simulink model "xEMU_SimulationModel3_rule1"  (R2017b)
settings: Solver=ode4  StartTime=0.0  StopTime=8192  FixedStep=0.01  RelTol=1e-3
undefined symbols (not defined in the file): a1, a2, a3, a4, ACO, BAT, Battery, DCT, DRT, EMS, ENV, Fahrzyklus_VS_modell, height_BAT, leistung, lib_bat, Maximum, Maximum_position, Num_cells, P_FC_max_long, P_FC_min_long, P_FC_step_max, Pbat_charge_max, Pbat_discharge_max, Pfc_max, Pfc_min, SOC_tar, time_peaks, TRM, velocity_peaks
libraries: simulink x5
(part 13 of 15)

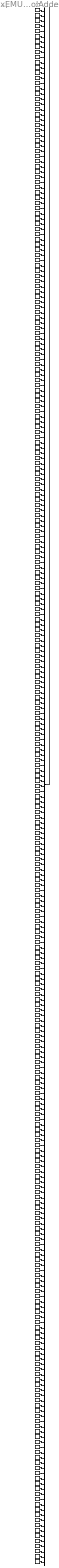
== system xEMU_SimulationModel3_rule1/Battery (BAT)_mittel/Subsystem1/Thermal/Coolings/CoolAdder ==
  P_cool : Inport
  Add_FV_{1..300} (300 alike) : Sum  Inputs=-
  Demux : Demux  Outputs=2
  Mux : Mux  Inputs=300
  P_FV : Outport
  wires:
  P_cool/1 -> Demux/1
  Mux/1 -> P_FV/1
  Add_FV_1/1 -> Mux/1
  Add_FV_2/1 -> Mux/2
  Add_FV_3/1 -> Mux/3
  Add_FV_4/1 -> Mux/4
  Add_FV_5/1 -> Mux/5
  Add_FV_6/1 -> Mux/6
  Add_FV_7/1 -> Mux/7
  Add_FV_8/1 -> Mux/8
  Add_FV_9/1 -> Mux/9
  Add_FV_10/1 -> Mux/10
  Add_FV_11/1 -> Mux/11
  Add_FV_12/1 -> Mux/12
  Add_FV_13/1 -> Mux/13
  Add_FV_14/1 -> Mux/14
  Add_FV_15/1 -> Mux/15
  Add_FV_16/1 -> Mux/16
  Add_FV_17/1 -> Mux/17
  Add_FV_18/1 -> Mux/18
  Add_FV_19/1 -> Mux/19
  Add_FV_20/1 -> Mux/20
  Add_FV_21/1 -> Mux/21
  Add_FV_22/1 -> Mux/22
  Add_FV_23/1 -> Mux/23
  Add_FV_24/1 -> Mux/24
  Add_FV_25/1 -> Mux/25
  Add_FV_26/1 -> Mux/26
  Add_FV_27/1 -> Mux/27
  Add_FV_28/1 -> Mux/28
  Add_FV_29/1 -> Mux/29
  Add_FV_30/1 -> Mux/30
  Add_FV_31/1 -> Mux/31
  Add_FV_32/1 -> Mux/32
  Add_FV_33/1 -> Mux/33
  Add_FV_34/1 -> Mux/34
  Add_FV_35/1 -> Mux/35
  Add_FV_36/1 -> Mux/36
  Add_FV_37/1 -> Mux/37
  Add_FV_38/1 -> Mux/38
  Add_FV_39/1 -> Mux/39
  Add_FV_40/1 -> Mux/40
  Add_FV_41/1 -> Mux/41
  Add_FV_42/1 -> Mux/42
  Add_FV_43/1 -> Mux/43
  Add_FV_44/1 -> Mux/44
  Add_FV_45/1 -> Mux/45
  Add_FV_46/1 -> Mux/46
  Add_FV_47/1 -> Mux/47
  Add_FV_48/1 -> Mux/48
  Add_FV_49/1 -> Mux/49
  Add_FV_50/1 -> Mux/50
  Add_FV_51/1 -> Mux/51
  Add_FV_52/1 -> Mux/52
  Add_FV_53/1 -> Mux/53
  Add_FV_54/1 -> Mux/54
  Add_FV_55/1 -> Mux/55
  Add_FV_56/1 -> Mux/56
  Add_FV_57/1 -> Mux/57
  Add_FV_58/1 -> Mux/58
  Add_FV_59/1 -> Mux/59
  Add_FV_60/1 -> Mux/60
  Add_FV_61/1 -> Mux/61
  Add_FV_62/1 -> Mux/62
  Add_FV_63/1 -> Mux/63
  Add_FV_64/1 -> Mux/64
  Add_FV_65/1 -> Mux/65
  Add_FV_66/1 -> Mux/66
  Add_FV_67/1 -> Mux/67
  Add_FV_68/1 -> Mux/68
  Add_FV_69/1 -> Mux/69
  Add_FV_70/1 -> Mux/70
  Add_FV_71/1 -> Mux/71
  Add_FV_72/1 -> Mux/72
  Add_FV_73/1 -> Mux/73
  Add_FV_74/1 -> Mux/74
  Add_FV_75/1 -> Mux/75
  Add_FV_76/1 -> Mux/76
  Add_FV_77/1 -> Mux/77
  Add_FV_78/1 -> Mux/78
  Add_FV_79/1 -> Mux/79
  Add_FV_80/1 -> Mux/80
  Add_FV_81/1 -> Mux/81
  Add_FV_82/1 -> Mux/82
  Add_FV_83/1 -> Mux/83
  Add_FV_84/1 -> Mux/84
  Add_FV_85/1 -> Mux/85
  Add_FV_86/1 -> Mux/86
  Add_FV_87/1 -> Mux/87
  Add_FV_88/1 -> Mux/88
  Add_FV_89/1 -> Mux/89
  Add_FV_90/1 -> Mux/90
  Add_FV_91/1 -> Mux/91
  Add_FV_92/1 -> Mux/92
  Add_FV_93/1 -> Mux/93
  Add_FV_94/1 -> Mux/94
  Add_FV_95/1 -> Mux/95
  Add_FV_96/1 -> Mux/96
  Add_FV_97/1 -> Mux/97
  Add_FV_98/1 -> Mux/98
  Add_FV_99/1 -> Mux/99
  Add_FV_100/1 -> Mux/100
  Add_FV_101/1 -> Mux/101
  Add_FV_102/1 -> Mux/102
  Add_FV_103/1 -> Mux/103
  Add_FV_104/1 -> Mux/104
  Add_FV_105/1 -> Mux/105
  Add_FV_106/1 -> Mux/106
  Add_FV_107/1 -> Mux/107
  Add_FV_108/1 -> Mux/108
  Add_FV_109/1 -> Mux/109
  Add_FV_110/1 -> Mux/110
  Add_FV_111/1 -> Mux/111
  Add_FV_112/1 -> Mux/112
  Add_FV_113/1 -> Mux/113
  Add_FV_114/1 -> Mux/114
  Add_FV_115/1 -> Mux/115
  Add_FV_116/1 -> Mux/116
  Add_FV_117/1 -> Mux/117
  Add_FV_118/1 -> Mux/118
  Add_FV_119/1 -> Mux/119
  Add_FV_120/1 -> Mux/120
  Add_FV_121/1 -> Mux/121
  Add_FV_122/1 -> Mux/122
  Add_FV_123/1 -> Mux/123
  Add_FV_124/1 -> Mux/124
  Add_FV_125/1 -> Mux/125
  Add_FV_126/1 -> Mux/126
  Add_FV_127/1 -> Mux/127
  Add_FV_128/1 -> Mux/128
  Add_FV_129/1 -> Mux/129
  Add_FV_130/1 -> Mux/130
  Add_FV_131/1 -> Mux/131
  Add_FV_132/1 -> Mux/132
  Add_FV_133/1 -> Mux/133
  Add_FV_134/1 -> Mux/134
  Add_FV_135/1 -> Mux/135
  Add_FV_136/1 -> Mux/136
  Add_FV_137/1 -> Mux/137
  Add_FV_138/1 -> Mux/138
  Add_FV_139/1 -> Mux/139
  Add_FV_140/1 -> Mux/140
  Add_FV_141/1 -> Mux/141
  Add_FV_142/1 -> Mux/142
  Add_FV_143/1 -> Mux/143
  Add_FV_144/1 -> Mux/144
  Add_FV_145/1 -> Mux/145
  Add_FV_146/1 -> Mux/146
  Add_FV_147/1 -> Mux/147
  Add_FV_148/1 -> Mux/148
  Add_FV_149/1 -> Mux/149
  Add_FV_150/1 -> Mux/150
  Add_FV_151/1 -> Mux/151
  Add_FV_152/1 -> Mux/152
  Add_FV_153/1 -> Mux/153
  Add_FV_154/1 -> Mux/154
  Add_FV_155/1 -> Mux/155
  Add_FV_156/1 -> Mux/156
  Add_FV_157/1 -> Mux/157
  Add_FV_158/1 -> Mux/158
  Add_FV_159/1 -> Mux/159
  Add_FV_160/1 -> Mux/160
  Add_FV_161/1 -> Mux/161
  Add_FV_162/1 -> Mux/162
  Add_FV_163/1 -> Mux/163
  Add_FV_164/1 -> Mux/164
  Add_FV_165/1 -> Mux/165
  Add_FV_166/1 -> Mux/166
  Add_FV_167/1 -> Mux/167
  Add_FV_168/1 -> Mux/168
  Add_FV_169/1 -> Mux/169
  Add_FV_170/1 -> Mux/170
  Add_FV_171/1 -> Mux/171
  Add_FV_172/1 -> Mux/172
  Add_FV_173/1 -> Mux/173
  Add_FV_174/1 -> Mux/174
  Add_FV_175/1 -> Mux/175
  Add_FV_176/1 -> Mux/176
  Add_FV_177/1 -> Mux/177
  Add_FV_178/1 -> Mux/178
  Add_FV_179/1 -> Mux/179
  Add_FV_180/1 -> Mux/180
  Add_FV_181/1 -> Mux/181
  Add_FV_182/1 -> Mux/182
  Add_FV_183/1 -> Mux/183
  Add_FV_184/1 -> Mux/184
  Add_FV_185/1 -> Mux/185
  Add_FV_186/1 -> Mux/186
  Add_FV_187/1 -> Mux/187
  Add_FV_188/1 -> Mux/188
  Add_FV_189/1 -> Mux/189
  Add_FV_190/1 -> Mux/190
  Add_FV_191/1 -> Mux/191
  Add_FV_192/1 -> Mux/192
  Add_FV_193/1 -> Mux/193
  Add_FV_194/1 -> Mux/194
  Add_FV_195/1 -> Mux/195
  Add_FV_196/1 -> Mux/196
  Add_FV_197/1 -> Mux/197
  Add_FV_198/1 -> Mux/198
  Add_FV_199/1 -> Mux/199
  Add_FV_200/1 -> Mux/200
  Add_FV_201/1 -> Mux/201
  Add_FV_202/1 -> Mux/202
  Add_FV_203/1 -> Mux/203
  Add_FV_204/1 -> Mux/204
  Add_FV_205/1 -> Mux/205
  Add_FV_206/1 -> Mux/206
  Add_FV_207/1 -> Mux/207
  Add_FV_208/1 -> Mux/208
  Add_FV_209/1 -> Mux/209
  Add_FV_210/1 -> Mux/210
  Add_FV_211/1 -> Mux/211
  Add_FV_212/1 -> Mux/212
  Add_FV_213/1 -> Mux/213
  Add_FV_214/1 -> Mux/214
  Add_FV_215/1 -> Mux/215
  Add_FV_216/1 -> Mux/216
  Add_FV_217/1 -> Mux/217
  Add_FV_218/1 -> Mux/218
  Add_FV_219/1 -> Mux/219
  Add_FV_220/1 -> Mux/220
  Add_FV_221/1 -> Mux/221
  Add_FV_222/1 -> Mux/222
  Add_FV_223/1 -> Mux/223
  Add_FV_224/1 -> Mux/224
  Add_FV_225/1 -> Mux/225
  Add_FV_226/1 -> Mux/226
  Add_FV_227/1 -> Mux/227
  Add_FV_228/1 -> Mux/228
  Add_FV_229/1 -> Mux/229
  Add_FV_230/1 -> Mux/230
  Add_FV_231/1 -> Mux/231
  Add_FV_232/1 -> Mux/232
  Add_FV_233/1 -> Mux/233
  Add_FV_234/1 -> Mux/234
  Add_FV_235/1 -> Mux/235
  Add_FV_236/1 -> Mux/236
  Add_FV_237/1 -> Mux/237
  Add_FV_238/1 -> Mux/238
  Add_FV_239/1 -> Mux/239
  Add_FV_240/1 -> Mux/240
  Add_FV_241/1 -> Mux/241
  Add_FV_242/1 -> Mux/242
  Add_FV_243/1 -> Mux/243
  Add_FV_244/1 -> Mux/244
  Add_FV_245/1 -> Mux/245
  Add_FV_246/1 -> Mux/246
  Add_FV_247/1 -> Mux/247
  Add_FV_248/1 -> Mux/248
  Add_FV_249/1 -> Mux/249
  Add_FV_250/1 -> Mux/250
  Add_FV_251/1 -> Mux/251
  Add_FV_252/1 -> Mux/252
  Add_FV_253/1 -> Mux/253
  Add_FV_254/1 -> Mux/254
  Add_FV_255/1 -> Mux/255
  Add_FV_256/1 -> Mux/256
  Add_FV_257/1 -> Mux/257
  Add_FV_258/1 -> Mux/258
  Add_FV_259/1 -> Mux/259
  Add_FV_260/1 -> Mux/260
  Add_FV_261/1 -> Mux/261
  Add_FV_262/1 -> Mux/262
  Add_FV_263/1 -> Mux/263
  Add_FV_264/1 -> Mux/264
  Add_FV_265/1 -> Mux/265
  Add_FV_266/1 -> Mux/266
  Add_FV_267/1 -> Mux/267
  Add_FV_268/1 -> Mux/268
  Add_FV_269/1 -> Mux/269
  Add_FV_270/1 -> Mux/270
  Add_FV_271/1 -> Mux/271
  Add_FV_272/1 -> Mux/272
  Add_FV_273/1 -> Mux/273
  Add_FV_274/1 -> Mux/274
  Add_FV_275/1 -> Mux/275
  Add_FV_276/1 -> Mux/276
  Add_FV_277/1 -> Mux/277
  Add_FV_278/1 -> Mux/278
  Add_FV_279/1 -> Mux/279
  Add_FV_280/1 -> Mux/280
  Add_FV_281/1 -> Mux/281
  Add_FV_282/1 -> Mux/282
  Add_FV_283/1 -> Mux/283
  Add_FV_284/1 -> Mux/284
  Add_FV_285/1 -> Mux/285
  Add_FV_286/1 -> Mux/286
  Add_FV_287/1 -> Mux/287
  Add_FV_288/1 -> Mux/288
  Add_FV_289/1 -> Mux/289
  Add_FV_290/1 -> Mux/290
  Add_FV_291/1 -> Mux/291
  Add_FV_292/1 -> Mux/292
  Add_FV_293/1 -> Mux/293
  Add_FV_294/1 -> Mux/294
  Add_FV_295/1 -> Mux/295
  Add_FV_296/1 -> Mux/296
  Add_FV_297/1 -> Mux/297
  Add_FV_298/1 -> Mux/298
  Add_FV_299/1 -> Mux/299
  Add_FV_300/1 -> Mux/300

== system xEMU_SimulationModel3_rule1/Battery (BAT)_mittel_02/Cell/ElectricalCircuit/SerialTwoPort_Elem1/Cellelement_Elem1 ==
  OhmicResistance_Elem4 : Subsystem
  ParallelRC_Elem1 : Subsystem
  ParallelRC_Elem2 : Subsystem
  ParallelRC_Elem3 : Subsystem
  SoC : Integrator  ExternalReset=rising  InitialCondition=SOC_tar*100  LimitOutput=on  UpperSaturationLimit=100  LowerSaturationLimit=0
  SoCFactor : Gain  Gain=0.0012077
  VoltageSource_Elem5 : Subsystem
  tag scope: SoC_CellElement1=global
  wires:
  [Reset] -> SoC/2
  SoC/1 -> OhmicResistance_Elem4/2(SoC), VoltageSource_Elem5/2(SoC), ParallelRC_Elem3/2(SoC), ParallelRC_Elem2/2(SoC), ParallelRC_Elem1/2(SoC), [SoC_CellElement1]
  [I_CellElement1] -> SoCFactor/1
  SoCFactor/1 -> SoC/1
  [T_CellElement1] -> OhmicResistance_Elem4/1(T), VoltageSource_Elem5/1(T), ParallelRC_Elem3/1(T), ParallelRC_Elem2/1(T), ParallelRC_Elem1/1(T)

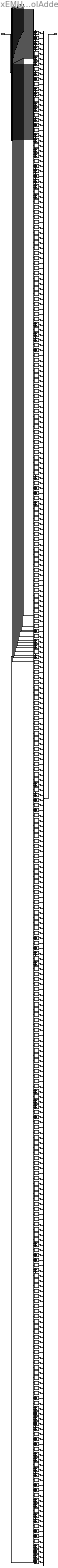
== system xEMU_SimulationModel3_rule1/Battery (BAT)_mittel_02/Cell/Thermal/Coolings/CoolAdder ==
  P_cool : Inport
  Add_FV_{1,3,28,30,271,273,298,300} (8 alike) : Sum  Inputs=+++
  Add_FV_{2,4,6..7,9..10,12..13,15..16,18..19,21..22,24..25,27,29,31,33,58,60..61,63,88,90..91,93,118,120..121,123,148,150..151,153,178,180..181,183,208,210..211,213,238,240..241,243,268,270,272,274,276..277,279..280,282..283,285..286,288..289,291..292,294..295,297,299} (68 alike) : Sum
  Add_FV_{5,8,11,14,17,20,23,26,32,34,36..37,39..40,42..43,45..46,48..49,51..52,54..55,57,59,62,64,66..67,69..70,72..73,75..76,78..79,81..82,84..85,87,89,92,94,96..97,99..100,102..103,105..106,108..109,111..112,114..115,117,119,122,124,126..127,129..130,132..133,135..136,138..139,141..142,144..145,147,149,152,154,156..157,159..160,162..163,165..166,168..169,171..172,174..175,177,179,182,184,186..187,189..190,192..193,195..196,198..199,201..202,204..205,207,209,212,214,216..217,219..220,222..223,225..226,228..229,231..232,234..235,237,239,242,244,246..247,249..250,252..253,255..256,258..259,261..262,264..265,267,269,275,278,281,284,287,290,293,296} (160 alike) : Sum  Inputs=+
  Add_FV_{35,38,41,44,47,50,53,56,65,68,71,74,77,80,83,86,95,98,101,104,107,110,113,116,125,128,131,134,137,140,143,146,155,158,161,164,167,170,173,176,185,188,191,194,197,200,203,206,215,218,221,224,227,230,233,236,245,248,251,254,257,260,263,266} (64 alike) : Sum  Inputs=-
  Demux : Demux  Outputs=320
  Mux : Mux  Inputs=300
  P_FV : Outport
  wires:
  P_cool/1 -> Demux/1
  Mux/1 -> P_FV/1
  Add_FV_1/1 -> Mux/1
  Add_FV_2/1 -> Mux/2
  Add_FV_3/1 -> Mux/3
  Add_FV_4/1 -> Mux/4
  Add_FV_5/1 -> Mux/5
  Add_FV_6/1 -> Mux/6
  Add_FV_7/1 -> Mux/7
  Add_FV_8/1 -> Mux/8
  Add_FV_9/1 -> Mux/9
  Add_FV_10/1 -> Mux/10
  Add_FV_11/1 -> Mux/11
  Add_FV_12/1 -> Mux/12
  Add_FV_13/1 -> Mux/13
  Add_FV_14/1 -> Mux/14
  Add_FV_15/1 -> Mux/15
  Add_FV_16/1 -> Mux/16
  Add_FV_17/1 -> Mux/17
  Add_FV_18/1 -> Mux/18
  Add_FV_19/1 -> Mux/19
  Add_FV_20/1 -> Mux/20
  Add_FV_21/1 -> Mux/21
  Add_FV_22/1 -> Mux/22
  Add_FV_23/1 -> Mux/23
  Add_FV_24/1 -> Mux/24
  Add_FV_25/1 -> Mux/25
  Add_FV_26/1 -> Mux/26
  Add_FV_27/1 -> Mux/27
  Add_FV_28/1 -> Mux/28
  Add_FV_29/1 -> Mux/29
  Add_FV_30/1 -> Mux/30
  Add_FV_31/1 -> Mux/31
  Add_FV_32/1 -> Mux/32
  Add_FV_33/1 -> Mux/33
  Add_FV_34/1 -> Mux/34
  Add_FV_35/1 -> Mux/35
  Add_FV_36/1 -> Mux/36
  Add_FV_37/1 -> Mux/37
  Add_FV_38/1 -> Mux/38
  Add_FV_39/1 -> Mux/39
  Add_FV_40/1 -> Mux/40
  Add_FV_41/1 -> Mux/41
  Add_FV_42/1 -> Mux/42
  Add_FV_43/1 -> Mux/43
  Add_FV_44/1 -> Mux/44
  Add_FV_45/1 -> Mux/45
  Add_FV_46/1 -> Mux/46
  Add_FV_47/1 -> Mux/47
  Add_FV_48/1 -> Mux/48
  Add_FV_49/1 -> Mux/49
  Add_FV_50/1 -> Mux/50
  Add_FV_51/1 -> Mux/51
  Add_FV_52/1 -> Mux/52
  Add_FV_53/1 -> Mux/53
  Add_FV_54/1 -> Mux/54
  Add_FV_55/1 -> Mux/55
  Add_FV_56/1 -> Mux/56
  Add_FV_57/1 -> Mux/57
  Add_FV_58/1 -> Mux/58
  Add_FV_59/1 -> Mux/59
  Add_FV_60/1 -> Mux/60
  Add_FV_61/1 -> Mux/61
  Add_FV_62/1 -> Mux/62
  Add_FV_63/1 -> Mux/63
  Add_FV_64/1 -> Mux/64
  Add_FV_65/1 -> Mux/65
  Add_FV_66/1 -> Mux/66
  Add_FV_67/1 -> Mux/67
  Add_FV_68/1 -> Mux/68
  Add_FV_69/1 -> Mux/69
  Add_FV_70/1 -> Mux/70
  Add_FV_71/1 -> Mux/71
  Add_FV_72/1 -> Mux/72
  Add_FV_73/1 -> Mux/73
  Add_FV_74/1 -> Mux/74
  Add_FV_75/1 -> Mux/75
  Add_FV_76/1 -> Mux/76
  Add_FV_77/1 -> Mux/77
  Add_FV_78/1 -> Mux/78
  Add_FV_79/1 -> Mux/79
  Add_FV_80/1 -> Mux/80
  Add_FV_81/1 -> Mux/81
  Add_FV_82/1 -> Mux/82
  Add_FV_83/1 -> Mux/83
  Add_FV_84/1 -> Mux/84
  Add_FV_85/1 -> Mux/85
  Add_FV_86/1 -> Mux/86
  Add_FV_87/1 -> Mux/87
  Add_FV_88/1 -> Mux/88
  Add_FV_89/1 -> Mux/89
  Add_FV_90/1 -> Mux/90
  Add_FV_91/1 -> Mux/91
  Add_FV_92/1 -> Mux/92
  Add_FV_93/1 -> Mux/93
  Add_FV_94/1 -> Mux/94
  Add_FV_95/1 -> Mux/95
  Add_FV_96/1 -> Mux/96
  Add_FV_97/1 -> Mux/97
  Add_FV_98/1 -> Mux/98
  Add_FV_99/1 -> Mux/99
  Add_FV_100/1 -> Mux/100
  Add_FV_101/1 -> Mux/101
  Add_FV_102/1 -> Mux/102
  Add_FV_103/1 -> Mux/103
  Add_FV_104/1 -> Mux/104
  Add_FV_105/1 -> Mux/105
  Add_FV_106/1 -> Mux/106
  Add_FV_107/1 -> Mux/107
  Add_FV_108/1 -> Mux/108
  Add_FV_109/1 -> Mux/109
  Add_FV_110/1 -> Mux/110
  Add_FV_111/1 -> Mux/111
  Add_FV_112/1 -> Mux/112
  Add_FV_113/1 -> Mux/113
  Add_FV_114/1 -> Mux/114
  Add_FV_115/1 -> Mux/115
  Add_FV_116/1 -> Mux/116
  Add_FV_117/1 -> Mux/117
  Add_FV_118/1 -> Mux/118
  Add_FV_119/1 -> Mux/119
  Add_FV_120/1 -> Mux/120
  Add_FV_121/1 -> Mux/121
  Add_FV_122/1 -> Mux/122
  Add_FV_123/1 -> Mux/123
  Add_FV_124/1 -> Mux/124
  Add_FV_125/1 -> Mux/125
  Add_FV_126/1 -> Mux/126
  Add_FV_127/1 -> Mux/127
  Add_FV_128/1 -> Mux/128
  Add_FV_129/1 -> Mux/129
  Add_FV_130/1 -> Mux/130
  Add_FV_131/1 -> Mux/131
  Add_FV_132/1 -> Mux/132
  Add_FV_133/1 -> Mux/133
  Add_FV_134/1 -> Mux/134
  Add_FV_135/1 -> Mux/135
  Add_FV_136/1 -> Mux/136
  Add_FV_137/1 -> Mux/137
  Add_FV_138/1 -> Mux/138
  Add_FV_139/1 -> Mux/139
  Add_FV_140/1 -> Mux/140
  Add_FV_141/1 -> Mux/141
  Add_FV_142/1 -> Mux/142
  Add_FV_143/1 -> Mux/143
  Add_FV_144/1 -> Mux/144
  Add_FV_145/1 -> Mux/145
  Add_FV_146/1 -> Mux/146
  Add_FV_147/1 -> Mux/147
  Add_FV_148/1 -> Mux/148
  Add_FV_149/1 -> Mux/149
  Add_FV_150/1 -> Mux/150
  Add_FV_151/1 -> Mux/151
  Add_FV_152/1 -> Mux/152
  Add_FV_153/1 -> Mux/153
  Add_FV_154/1 -> Mux/154
  Add_FV_155/1 -> Mux/155
  Add_FV_156/1 -> Mux/156
  Add_FV_157/1 -> Mux/157
  Add_FV_158/1 -> Mux/158
  Add_FV_159/1 -> Mux/159
  Add_FV_160/1 -> Mux/160
  Add_FV_161/1 -> Mux/161
  Add_FV_162/1 -> Mux/162
  Add_FV_163/1 -> Mux/163
  Add_FV_164/1 -> Mux/164
  Add_FV_165/1 -> Mux/165
  Add_FV_166/1 -> Mux/166
  Add_FV_167/1 -> Mux/167
  Add_FV_168/1 -> Mux/168
  Add_FV_169/1 -> Mux/169
  Add_FV_170/1 -> Mux/170
  Add_FV_171/1 -> Mux/171
  Add_FV_172/1 -> Mux/172
  Add_FV_173/1 -> Mux/173
  Add_FV_174/1 -> Mux/174
  Add_FV_175/1 -> Mux/175
  Add_FV_176/1 -> Mux/176
  Add_FV_177/1 -> Mux/177
  Add_FV_178/1 -> Mux/178
  Add_FV_179/1 -> Mux/179
  Add_FV_180/1 -> Mux/180
  Add_FV_181/1 -> Mux/181
  Add_FV_182/1 -> Mux/182
  Add_FV_183/1 -> Mux/183
  Add_FV_184/1 -> Mux/184
  Add_FV_185/1 -> Mux/185
  Add_FV_186/1 -> Mux/186
  Add_FV_187/1 -> Mux/187
  Add_FV_188/1 -> Mux/188
  Add_FV_189/1 -> Mux/189
  Add_FV_190/1 -> Mux/190
  Add_FV_191/1 -> Mux/191
  Add_FV_192/1 -> Mux/192
  Add_FV_193/1 -> Mux/193
  Add_FV_194/1 -> Mux/194
  Add_FV_195/1 -> Mux/195
  Add_FV_196/1 -> Mux/196
  Add_FV_197/1 -> Mux/197
  Add_FV_198/1 -> Mux/198
  Add_FV_199/1 -> Mux/199
  Add_FV_200/1 -> Mux/200
  Add_FV_201/1 -> Mux/201
  Add_FV_202/1 -> Mux/202
  Add_FV_203/1 -> Mux/203
  Add_FV_204/1 -> Mux/204
  Add_FV_205/1 -> Mux/205
  Add_FV_206/1 -> Mux/206
  Add_FV_207/1 -> Mux/207
  Add_FV_208/1 -> Mux/208
  Add_FV_209/1 -> Mux/209
  Add_FV_210/1 -> Mux/210
  Add_FV_211/1 -> Mux/211
  Add_FV_212/1 -> Mux/212
  Add_FV_213/1 -> Mux/213
  Add_FV_214/1 -> Mux/214
  Add_FV_215/1 -> Mux/215
  Add_FV_216/1 -> Mux/216
  Add_FV_217/1 -> Mux/217
  Add_FV_218/1 -> Mux/218
  Add_FV_219/1 -> Mux/219
  Add_FV_220/1 -> Mux/220
  Add_FV_221/1 -> Mux/221
  Add_FV_222/1 -> Mux/222
  Add_FV_223/1 -> Mux/223
  Add_FV_224/1 -> Mux/224
  Add_FV_225/1 -> Mux/225
  Add_FV_226/1 -> Mux/226
  Add_FV_227/1 -> Mux/227
  Add_FV_228/1 -> Mux/228
  Add_FV_229/1 -> Mux/229
  Add_FV_230/1 -> Mux/230
  Add_FV_231/1 -> Mux/231
  Add_FV_232/1 -> Mux/232
  Add_FV_233/1 -> Mux/233
  Add_FV_234/1 -> Mux/234
  Add_FV_235/1 -> Mux/235
  Add_FV_236/1 -> Mux/236
  Add_FV_237/1 -> Mux/237
  Add_FV_238/1 -> Mux/238
  Add_FV_239/1 -> Mux/239
  Add_FV_240/1 -> Mux/240
  Add_FV_241/1 -> Mux/241
  Add_FV_242/1 -> Mux/242
  Add_FV_243/1 -> Mux/243
  Add_FV_244/1 -> Mux/244
  Add_FV_245/1 -> Mux/245
  Add_FV_246/1 -> Mux/246
  Add_FV_247/1 -> Mux/247
  Add_FV_248/1 -> Mux/248
  Add_FV_249/1 -> Mux/249
  Add_FV_250/1 -> Mux/250
  Add_FV_251/1 -> Mux/251
  Add_FV_252/1 -> Mux/252
  Add_FV_253/1 -> Mux/253
  Add_FV_254/1 -> Mux/254
  Add_FV_255/1 -> Mux/255
  Add_FV_256/1 -> Mux/256
  Add_FV_257/1 -> Mux/257
  Add_FV_258/1 -> Mux/258
  Add_FV_259/1 -> Mux/259
  Add_FV_260/1 -> Mux/260
  Add_FV_261/1 -> Mux/261
  Add_FV_262/1 -> Mux/262
  Add_FV_263/1 -> Mux/263
  Add_FV_264/1 -> Mux/264
  Add_FV_265/1 -> Mux/265
  Add_FV_266/1 -> Mux/266
  Add_FV_267/1 -> Mux/267
  Add_FV_268/1 -> Mux/268
  Add_FV_269/1 -> Mux/269
  Add_FV_270/1 -> Mux/270
  Add_FV_271/1 -> Mux/271
  Add_FV_272/1 -> Mux/272
  Add_FV_273/1 -> Mux/273
  Add_FV_274/1 -> Mux/274
  Add_FV_275/1 -> Mux/275
  Add_FV_276/1 -> Mux/276
  Add_FV_277/1 -> Mux/277
  Add_FV_278/1 -> Mux/278
  Add_FV_279/1 -> Mux/279
  Add_FV_280/1 -> Mux/280
  Add_FV_281/1 -> Mux/281
  Add_FV_282/1 -> Mux/282
  Add_FV_283/1 -> Mux/283
  Add_FV_284/1 -> Mux/284
  Add_FV_285/1 -> Mux/285
  Add_FV_286/1 -> Mux/286
  Add_FV_287/1 -> Mux/287
  Add_FV_288/1 -> Mux/288
  Add_FV_289/1 -> Mux/289
  Add_FV_290/1 -> Mux/290
  Add_FV_291/1 -> Mux/291
  Add_FV_292/1 -> Mux/292
  Add_FV_293/1 -> Mux/293
  Add_FV_294/1 -> Mux/294
  Add_FV_295/1 -> Mux/295
  Add_FV_296/1 -> Mux/296
  Add_FV_297/1 -> Mux/297
  Add_FV_298/1 -> Mux/298
  Add_FV_299/1 -> Mux/299
  Add_FV_300/1 -> Mux/300
  Demux/1 -> Add_FV_1/1
  Demux/2 -> Add_FV_1/2
  Demux/3 -> Add_FV_1/3
  Demux/4 -> Add_FV_2/1
  Demux/5 -> Add_FV_2/2
  Demux/6 -> Add_FV_3/1
  Demux/7 -> Add_FV_3/2
  Demux/8 -> Add_FV_3/3
  Demux/9 -> Add_FV_4/1
  Demux/10 -> Add_FV_4/2
  Demux/11 -> Add_FV_5/1
  Demux/12 -> Add_FV_6/1
  Demux/13 -> Add_FV_6/2
  Demux/14 -> Add_FV_7/1
  Demux/15 -> Add_FV_7/2
  Demux/16 -> Add_FV_8/1
  Demux/17 -> Add_FV_9/1
  Demux/18 -> Add_FV_9/2
  Demux/19 -> Add_FV_10/1
  Demux/20 -> Add_FV_10/2
  Demux/21 -> Add_FV_11/1
  Demux/22 -> Add_FV_12/1
  Demux/23 -> Add_FV_12/2
  Demux/24 -> Add_FV_13/1
  Demux/25 -> Add_FV_13/2
  Demux/26 -> Add_FV_14/1
  Demux/27 -> Add_FV_15/1
  Demux/28 -> Add_FV_15/2
  Demux/29 -> Add_FV_16/1
  Demux/30 -> Add_FV_16/2
  Demux/31 -> Add_FV_17/1
  Demux/32 -> Add_FV_18/1
  Demux/33 -> Add_FV_18/2
  Demux/34 -> Add_FV_19/1
  Demux/35 -> Add_FV_19/2
  Demux/36 -> Add_FV_20/1
  Demux/37 -> Add_FV_21/1
  Demux/38 -> Add_FV_21/2
  Demux/39 -> Add_FV_22/1
  Demux/40 -> Add_FV_22/2
  Demux/41 -> Add_FV_23/1
  Demux/42 -> Add_FV_24/1
  Demux/43 -> Add_FV_24/2
  Demux/44 -> Add_FV_25/1
  Demux/45 -> Add_FV_25/2
  Demux/46 -> Add_FV_26/1
  Demux/47 -> Add_FV_27/1
  Demux/48 -> Add_FV_27/2
  Demux/49 -> Add_FV_28/1
  Demux/50 -> Add_FV_28/2
  Demux/51 -> Add_FV_28/3
  Demux/52 -> Add_FV_29/1
  Demux/53 -> Add_FV_29/2
  Demux/54 -> Add_FV_30/1
  Demux/55 -> Add_FV_30/2
  Demux/56 -> Add_FV_30/3
  Demux/57 -> Add_FV_31/1
  Demux/58 -> Add_FV_31/2
  Demux/59 -> Add_FV_32/1
  Demux/60 -> Add_FV_33/1
  Demux/61 -> Add_FV_33/2
  Demux/62 -> Add_FV_34/1
  Demux/63 -> Add_FV_36/1
  Demux/64 -> Add_FV_37/1
  Demux/65 -> Add_FV_39/1
  Demux/66 -> Add_FV_40/1
  Demux/67 -> Add_FV_42/1
  Demux/68 -> Add_FV_43/1
  Demux/69 -> Add_FV_45/1
  Demux/70 -> Add_FV_46/1
  Demux/71 -> Add_FV_48/1
  Demux/72 -> Add_FV_49/1
  Demux/73 -> Add_FV_51/1
  Demux/74 -> Add_FV_52/1
  Demux/75 -> Add_FV_54/1
  Demux/76 -> Add_FV_55/1
  Demux/77 -> Add_FV_57/1
  Demux/78 -> Add_FV_58/1
  Demux/79 -> Add_FV_58/2
  Demux/80 -> Add_FV_59/1
  Demux/81 -> Add_FV_60/1
  Demux/82 -> Add_FV_60/2
  Demux/83 -> Add_FV_61/1
  Demux/84 -> Add_FV_61/2
  Demux/85 -> Add_FV_62/1
  Demux/86 -> Add_FV_63/1
  Demux/87 -> Add_FV_63/2
  Demux/88 -> Add_FV_64/1
  Demux/89 -> Add_FV_66/1
  Demux/90 -> Add_FV_67/1
  Demux/91 -> Add_FV_69/1
  Demux/92 -> Add_FV_70/1
  Demux/93 -> Add_FV_72/1
  Demux/94 -> Add_FV_73/1
  Demux/95 -> Add_FV_75/1
  Demux/96 -> Add_FV_76/1
  Demux/97 -> Add_FV_78/1
  Demux/98 -> Add_FV_79/1
  Demux/99 -> Add_FV_81/1
  Demux/100 -> Add_FV_82/1
  Demux/101 -> Add_FV_84/1
  Demux/102 -> Add_FV_85/1
  Demux/103 -> Add_FV_87/1
  Demux/104 -> Add_FV_88/1
  Demux/105 -> Add_FV_88/2
  Demux/106 -> Add_FV_89/1
  Demux/107 -> Add_FV_90/1
  Demux/108 -> Add_FV_90/2
  Demux/109 -> Add_FV_91/1
  Demux/110 -> Add_FV_91/2
  Demux/111 -> Add_FV_92/1
  Demux/112 -> Add_FV_93/1
  Demux/113 -> Add_FV_93/2
  Demux/114 -> Add_FV_94/1
  Demux/115 -> Add_FV_96/1
  Demux/116 -> Add_FV_97/1
  Demux/117 -> Add_FV_99/1
  Demux/118 -> Add_FV_100/1
  Demux/119 -> Add_FV_102/1
  Demux/120 -> Add_FV_103/1
  Demux/121 -> Add_FV_105/1
  Demux/122 -> Add_FV_106/1
  Demux/123 -> Add_FV_108/1
  Demux/124 -> Add_FV_109/1
  Demux/125 -> Add_FV_111/1
  Demux/126 -> Add_FV_112/1
  Demux/127 -> Add_FV_114/1
  Demux/128 -> Add_FV_115/1
  Demux/129 -> Add_FV_117/1
  Demux/130 -> Add_FV_118/1
  Demux/131 -> Add_FV_118/2
  Demux/132 -> Add_FV_119/1
  Demux/133 -> Add_FV_120/1
  Demux/134 -> Add_FV_120/2
  Demux/135 -> Add_FV_121/1
  Demux/136 -> Add_FV_121/2
  Demux/137 -> Add_FV_122/1
  Demux/138 -> Add_FV_123/1
  Demux/139 -> Add_FV_123/2
  Demux/140 -> Add_FV_124/1
  Demux/141 -> Add_FV_126/1
  Demux/142 -> Add_FV_127/1
  Demux/143 -> Add_FV_129/1
  Demux/144 -> Add_FV_130/1
  Demux/145 -> Add_FV_132/1
  Demux/146 -> Add_FV_133/1
  Demux/147 -> Add_FV_135/1
  Demux/148 -> Add_FV_136/1
  Demux/149 -> Add_FV_138/1
  Demux/150 -> Add_FV_139/1
  Demux/151 -> Add_FV_141/1
  Demux/152 -> Add_FV_142/1
  Demux/153 -> Add_FV_144/1
  Demux/154 -> Add_FV_145/1
  Demux/155 -> Add_FV_147/1
  Demux/156 -> Add_FV_148/1
  Demux/157 -> Add_FV_148/2
  Demux/158 -> Add_FV_149/1
  Demux/159 -> Add_FV_150/1
  Demux/160 -> Add_FV_150/2
  Demux/161 -> Add_FV_151/1
  Demux/162 -> Add_FV_151/2
  Demux/163 -> Add_FV_152/1
  Demux/164 -> Add_FV_153/1
  Demux/165 -> Add_FV_153/2
  Demux/166 -> Add_FV_154/1
  Demux/167 -> Add_FV_156/1
  Demux/168 -> Add_FV_157/1
  Demux/169 -> Add_FV_159/1
  Demux/170 -> Add_FV_160/1
  Demux/171 -> Add_FV_162/1
  Demux/172 -> Add_FV_163/1
  Demux/173 -> Add_FV_165/1
  Demux/174 -> Add_FV_166/1
  Demux/175 -> Add_FV_168/1
  Demux/176 -> Add_FV_169/1
  Demux/177 -> Add_FV_171/1
  Demux/178 -> Add_FV_172/1
  Demux/179 -> Add_FV_174/1
  Demux/180 -> Add_FV_175/1
  Demux/181 -> Add_FV_177/1
  Demux/182 -> Add_FV_178/1
  Demux/183 -> Add_FV_178/2
  Demux/184 -> Add_FV_179/1
  Demux/185 -> Add_FV_180/1
  Demux/186 -> Add_FV_180/2
  Demux/187 -> Add_FV_181/1
  Demux/188 -> Add_FV_181/2
  Demux/189 -> Add_FV_182/1
  Demux/190 -> Add_FV_183/1
  Demux/191 -> Add_FV_183/2
  Demux/192 -> Add_FV_184/1
  Demux/193 -> Add_FV_186/1
  Demux/194 -> Add_FV_187/1
  Demux/195 -> Add_FV_189/1
  Demux/196 -> Add_FV_190/1
  Demux/197 -> Add_FV_192/1
  Demux/198 -> Add_FV_193/1
  Demux/199 -> Add_FV_195/1
  Demux/200 -> Add_FV_196/1
  Demux/201 -> Add_FV_198/1
  Demux/202 -> Add_FV_199/1
  Demux/203 -> Add_FV_201/1
  Demux/204 -> Add_FV_202/1
  Demux/205 -> Add_FV_204/1
  Demux/206 -> Add_FV_205/1
  Demux/207 -> Add_FV_207/1
  Demux/208 -> Add_FV_208/1
  Demux/209 -> Add_FV_208/2
  Demux/210 -> Add_FV_209/1
  Demux/211 -> Add_FV_210/1
  Demux/212 -> Add_FV_210/2
  Demux/213 -> Add_FV_211/1
  Demux/214 -> Add_FV_211/2
  Demux/215 -> Add_FV_212/1
  Demux/216 -> Add_FV_213/1
  Demux/217 -> Add_FV_213/2
  Demux/218 -> Add_FV_214/1
  Demux/219 -> Add_FV_216/1
  Demux/220 -> Add_FV_217/1
  Demux/221 -> Add_FV_219/1
  Demux/222 -> Add_FV_220/1
  Demux/223 -> Add_FV_222/1
  Demux/224 -> Add_FV_223/1
  Demux/225 -> Add_FV_225/1
  Demux/226 -> Add_FV_226/1
  Demux/227 -> Add_FV_228/1
  Demux/228 -> Add_FV_229/1
  Demux/229 -> Add_FV_231/1
  Demux/230 -> Add_FV_232/1
  Demux/231 -> Add_FV_234/1
  Demux/232 -> Add_FV_235/1
  Demux/233 -> Add_FV_237/1
  Demux/234 -> Add_FV_238/1
  Demux/235 -> Add_FV_238/2
  Demux/236 -> Add_FV_239/1
  Demux/237 -> Add_FV_240/1
  Demux/238 -> Add_FV_240/2
  Demux/239 -> Add_FV_241/1
  Demux/240 -> Add_FV_241/2
  Demux/241 -> Add_FV_242/1
  Demux/242 -> Add_FV_243/1
  Demux/243 -> Add_FV_243/2
  Demux/244 -> Add_FV_244/1
  Demux/245 -> Add_FV_246/1
  Demux/246 -> Add_FV_247/1
  Demux/247 -> Add_FV_249/1
  Demux/248 -> Add_FV_250/1
  Demux/249 -> Add_FV_252/1
  Demux/250 -> Add_FV_253/1
  Demux/251 -> Add_FV_255/1
  Demux/252 -> Add_FV_256/1
  Demux/253 -> Add_FV_258/1
  Demux/254 -> Add_FV_259/1
  Demux/255 -> Add_FV_261/1
  Demux/256 -> Add_FV_262/1
  Demux/257 -> Add_FV_264/1
  Demux/258 -> Add_FV_265/1
  Demux/259 -> Add_FV_267/1
  Demux/260 -> Add_FV_268/1
  Demux/261 -> Add_FV_268/2
  Demux/262 -> Add_FV_269/1
  Demux/263 -> Add_FV_270/1
  Demux/264 -> Add_FV_270/2
  Demux/265 -> Add_FV_271/1
  Demux/266 -> Add_FV_271/2
  Demux/267 -> Add_FV_271/3
  Demux/268 -> Add_FV_272/1
  Demux/269 -> Add_FV_272/2
  Demux/270 -> Add_FV_273/1
  Demux/271 -> Add_FV_273/2
  Demux/272 -> Add_FV_273/3
  Demux/273 -> Add_FV_274/1
  Demux/274 -> Add_FV_274/2
  Demux/275 -> Add_FV_275/1
  Demux/276 -> Add_FV_276/1
  Demux/277 -> Add_FV_276/2
  Demux/278 -> Add_FV_277/1
  Demux/279 -> Add_FV_277/2
  Demux/280 -> Add_FV_278/1
  Demux/281 -> Add_FV_279/1
  Demux/282 -> Add_FV_279/2
  Demux/283 -> Add_FV_280/1
  Demux/284 -> Add_FV_280/2
  Demux/285 -> Add_FV_281/1
  Demux/286 -> Add_FV_282/1
  Demux/287 -> Add_FV_282/2
  Demux/288 -> Add_FV_283/1
  Demux/289 -> Add_FV_283/2
  Demux/290 -> Add_FV_284/1
  Demux/291 -> Add_FV_285/1
  Demux/292 -> Add_FV_285/2
  Demux/293 -> Add_FV_286/1
  Demux/294 -> Add_FV_286/2
  Demux/295 -> Add_FV_287/1
  Demux/296 -> Add_FV_288/1
  Demux/297 -> Add_FV_288/2
  Demux/298 -> Add_FV_289/1
  Demux/299 -> Add_FV_289/2
  Demux/300 -> Add_FV_290/1
  Demux/301 -> Add_FV_291/1
  Demux/302 -> Add_FV_291/2
  Demux/303 -> Add_FV_292/1
  Demux/304 -> Add_FV_292/2
  Demux/305 -> Add_FV_293/1
  Demux/306 -> Add_FV_294/1
  Demux/307 -> Add_FV_294/2
  Demux/308 -> Add_FV_295/1
  Demux/309 -> Add_FV_295/2
  Demux/310 -> Add_FV_296/1
  Demux/311 -> Add_FV_297/1
  Demux/312 -> Add_FV_297/2
  Demux/313 -> Add_FV_298/1
  Demux/314 -> Add_FV_298/2
  Demux/315 -> Add_FV_298/3
  Demux/316 -> Add_FV_299/1
  Demux/317 -> Add_FV_299/2
  Demux/318 -> Add_FV_300/1
  Demux/319 -> Add_FV_300/2
  Demux/320 -> Add_FV_300/3

== system xEMU_SimulationModel3_rule1/Battery (BAT)_mittel_02/Cell/Thermal/Coolings/DefaultCooling_Elem1 ==
  T_FV : Inport
  Add : Sum
  Add1 : Sum
  Areas : Gain  Gain=[8.50666666666667e-05;7.77333333333333e-05;0.00012296;8.50666666666667e-05;7.77333333333333e-05;8.50666666666667e-05;7.77333333333333e-05;0.00012296;8.50666666666667e-05;0.00012296;8.50666666666667e-05;8.50666666666667e-05;0.00012296;8.50666666666667e-05;0.00012296;8.50666666666667e-05;8.50666666666667e-05;0.00012296;8.50666666666667e-05;0.00012296;8.50666666666667e-05;8.50666666666667e-05;0.00012296;8.50666666666667e-05;0.00012296;8.50666666666667e-05;8.50666666666667e-05;0.00012296;8.50666666666667e-05;0.00012296;8.50666666666667e-05;8.50666666666667e-05;0.00012296;8.50666666666667e-05;0.00012296;8.50666666666667e-05;8.50666666666667e-05;0.00012296;8.50666666666667e-05;0.00012296;8.50666666666667e-05;8.50666666666667e-05;0.00012296;8.50666666666667e-05;0.00012296;8.50666666666667e-05;8.50666666666667e-05;0.00012296;8.50666666666667e-05;7.77333333333333e-05;0.00012296;8.50666666666667e-05;7.77333333333333e-05;8.50666666666667e-05;7.77333333333333e-05;0.00012296;7.77333333333333e-05;0.00012296;7.77333333333333e-05;7.77333333333333e-05;0.00012296;0.00012296;0.00012296;0.00012296;0.00012296;0.00012296;0.00012296;0.00012296;0.00012296;0.00012296;0.00012296;0.00012296;0.00012296;0.00012296;0.00012296;0.00012296;0.00012296;7.77333333333333e-05;0.00012296;7.77333333333333e-05;7.77333333333333e-05;0.00012296;7.77333333333333e-05;0.00012296;7.77333333333333e-05;7.77333333333333e-05;0.00012296;0.00012296;0.00012296;0.00012296;0.00012296;0.00012296;0.00012296;0.00012296;0.00012296;0.00012296;0.00012296;0.00012296;0.00012296;0.00012296;0.00012296;0.00012296;0.00012296;7.77333333333333e-05;0.00012296;7.77333333333333e-05;7.77333333333333e-05;0.00012296;7.77333333333333e-05;0.00012296;7.77333333333333e-05;7.77333333333333e-05;0.00012296;0.00012296;0.00012296;0.00012296;0.00012296;0.00012296;0.00012296;0.00012296;0.00012296;0.00012296;0.00012296;0.00012296;0.00012296;0.00012296;0.00012296;0.00012296;0.00012296;7.77333333333333e-05;0.00012296;7.77333333333333e-05;7.77333333333333e-05;0.00012296;7.77333333333333e-05;0.00012296;7.77333333333333e-05;7.77333333333333e-05;0.00012296;0.00012296;0.00012296;0.00012296;0.00012296;0.00012296;0.00012296;0.00012296;0.00012296;0.00012296;0.00012296;0.00012296;0.00012296;0.00012296;0.00012296;0.00012296;0.00012296;7.77333333333333e-05;0.00012296;7.77333333333333e-05;7.77333333333333e-05;0.00012296;7.77333333333333e-05;0.00012296;7.77333333333333e-05;7.77333333333333e-05;0.00012296;0.00012296;0.00012296;0.00012296;0.00012296;0.00012296;0.00012296;0.00012296;0.00012296;0.00012296;0.00012296;0.00012296;0.00012296;0.00012296;0.00012296;0.00012296;0.00012296;7.77333333333333e-05;0.00012296;7.77333333333333e-05;7.77333333333333e-05;0.00012296;7.77333333333333e-05;0.00012296;7.77333333333333e-05;7.77333333333333e-05;0.00012296;0.00012296;0.00012296;0.00012296;0.00012296;0.00012296;0.00012296;0.00012296;0.00012296;0.00012296;0.00012296;0.00012296;0.00012296;0.00012296;0.00012296;0.00012296;0.00012296;7.77333333333333e-05;0.00012296;7.77333333333333e-05;7.77333333333333e-05;0.00012296;7.77333333333333e-05;0.00012296;7.77333333333333e-05;7.77333333333333e-05;0.00012296;0.00012296;0.00012296;0.00012296;0.00012296;0.00012296;0.00012296;0.00012296;0.00012296;0.00012296;0.00012296;0.00012296;0.00012296;0.00012296;0.00012296;0.00012296;0.00012296;7.77333333333333e-05;0.00012296;7.77333333333333e-05;7.77333333333333e-05;0.00012296;7.77333333333333e-05;0.00012296;7.77333333333333e-05;7.77333333333333e-05;0.00012296;0.00012296;0.00012296;0.00012296;0.00012296;0.00012296;0.00012296;0.00012296;0.00012296;0.00012296;0.00012296;0.00012296;0.00012296;0.00012296;0.00012296;0.00012296;0.00012296;7.77333333333333e-05;0.00012296;7.77333333333333e-05;7.77333333333333e-05;0.00012296;8.50666666666667e-05;7.77333333333333e-05;0.00012296;8.50666666666667e-05;7.77333333333333e-05;8.50666666666667e-05;7.77333333333333e-05;0.00012296;8.50666666666667e-05;0.00012296;8.50666666666667e-05;8.50666666666667e-05;0.00012296;8.50666666666667e-05 ...(+722 chars)]
  CelsiusToKelvin : Constant  Value=273.15
  DefaultCooling : MATLAB Function  TreatAsAtomicUnit=on
  Selector : Selector  InputPortWidth=300  IndexOptions=Index vector (dialog)  Indices=[1 1 1 2 2 3 3 3 4 4 5 6 6 7 7 8 9 9 10 10 11 12 12 13 13 14 15 15 16 16 17 18 18 19 19 20 21 21 22 22 23 24 24 25 25 26 27 27 28 28 28 29 29 30 30 30 31 31 32 33 33 34 36 37 39 40 42 43 45 46 48 49 51 52 54 55 57 58 58 59 60 60 61 61 62 63 63 64 66 67 69 70 72 73 75 76 78 79 81 82 84 85 87 88 88 89 90 90 91 91 92 93 93 94 96 97 99 100 102 103 105 106 108 109 111 112 114 115 117 118 118 119 120 120 121 121 122 123 123 124 126 127 129 130 132 133 135 136 138 139 141 142 144 145 147 148 148 149 150 150 151 151 152 153 153 154 156 157 159 160 162 163 165 166 168 169 171 172 174 175 177 178 178 179 180 180 181 181 182 183 183 184 186 187 189 190 192 193 195 196 198 199 201 202 204 205 207 208 208 209 210 210 211 211 212 213 213 214 216 217 219 220 222 223 225 226 228 229 231 232 234 235 237 238 238 239 240 240 241 241 242 243 243 244 246 247 249 250 252 253 255 256 258 259 261 262 264 265 267 268 268 269 270 270 271 271 271 272 272 273 273 273 274 274 275 276 276 277 277 278 279 279 280 280 281 282 282 283 283 284 285 285 286 286 287 288 288 289 289 290 291 291 292 292 293 294 294 295 295 296 297 297 298 298 298 299 299 300 300 300]  OutputSizes=1
  P_cool : Outport
  wires:
  [AirTemperature] -> Add1/2
  Add1/1 -> DefaultCooling/2(airTemperature)
  CelsiusToKelvin/1 -> Add/2, Add1/1
  Areas/1 -> P_cool/1
  DefaultCooling/1(y) -> Areas/1
  Add/1 -> DefaultCooling/1(u)
  Selector/1 -> Add/1
  T_FV/1 -> Selector/1

== system xEMU_SimulationModel3_rule1/Drive Train (DRT)/Slipmodel and Traction /Variant Subsystem1/Mit_Schlupf_nach_Kalker/Slip Model ==
  note: gradient of tangential stress
  note: Tangential Force Fx=2*Fz*u/pi*(E/(1+E^2)+atan(E))
      |
      | gradient of tangential stress E=G*pi*a*b*C11*S/Fz/u/4
  Fz_tire : Inport
  slip : Inport  Port=2
  adhesion : Inport  Port=3
  " " : Fcn  Expr=u/(1+u^2)+atan(u)
  Divide : Product  Inputs=/*/
  Gain : Gain  Gain=Schub_drt*pi*a_drt*b_drt*C11_drt/4
  Gain1 : Gain  Gain=2/pi
  Product : Product  Inputs=3
  f_traction_tire : Outport
  wires:
  " "/1 -> Gain1/1
  Divide/1 -> " "/1
  Product/1 -> f_traction_tire/1
  Gain1/1 -> Product/2
  adhesion/1 -> Divide/3, Product/3
  Fz_tire/1 -> Divide/1, Product/1
  Gain/1 -> Divide/2
  slip/1 -> Gain/1

== system xEMU_SimulationModel3_rule1/Drive Train (DRT)/Slipmodel and Traction /Variant Subsystem1/Mit_Schlupf_nach_Kalker/Tire Dynamics ==
  Resistance of tire : Inport
  T_EMAdemandper_axis_Nm : Inport  Port=2
  v_train_m/s : Inport  Port=3
  Abs1 : Abs
  Abs2 : Abs
  Constant : Constant  Value=eps
  Gain : Gain  Gain=1/2
  Gain1 : Gain  Gain=1/J_drt
  Gain2 : Gain  Gain=R_wheel_drt_m
  Gain3 : Gain  Gain=1/50
  Integrator : Integrator  LowerSaturationLimit=0
  Integrator1 : Integrator
  MATLAB Function : MATLAB Function  TreatAsAtomicUnit=on
  MATLAB Function1 : MATLAB Function  TreatAsAtomicUnit=on
  Max : MinMax  Function=max  Inputs=3
  Product : Product
  Relay : Relay  OnSwitchValue=0.3  OffSwitchValue=0.01
  Relay1 : Relay  OnSwitchValue=0.2  OffSwitchValue=0.01
  Saturation : Saturate  UpperLimit=1  LowerLimit=-1
  Saturation2 : Saturate  UpperLimit=inf  LowerLimit=0
  Scope9 : Scope
  Subtract : Sum  Inputs=+-
  Subtract1 : Sum  Inputs=+-
  Sum : Sum  Inputs=-+|
  Switch : Switch  Criteria=u2 > Threshold
  slip : Outport
  WheelSpeed_rad/s : Outport  Port=2
  wires:
  MATLAB Function/1(s) -> Saturation/1
  Integrator/1 -> Saturation2/1  "ohneFilter"
  Constant/1 -> Max/3
  Abs2/1 -> Product/1, Max/2
  Abs1/1 -> Max/1
  Saturation/1 -> Switch/1  "Kalker"
  Sum/1 -> Gain1/1
  Max/1 -> MATLAB Function/2(v)
  Subtract/1 -> Subtract1/1, MATLAB Function/1(dv)
  Gain1/1 -> Integrator/1
  Gain2/1 -> Subtract/1, Abs1/1
  T_EMAdemandper_axis_Nm/1 -> Gain/1
  Gain/1 -> Sum/2
  Resistance of tire/1 -> Sum/1
  Product/1 -> Subtract1/2
  Subtract1/1 -> Gain3/1
  Gain3/1 -> Integrator1/1
  Integrator1/1 -> Switch/3, Product/2  "Dampf"
  Switch/1 -> slip/1
  v_train_m/s/1 -> Scope9/1, Relay1/1, Subtract/2, Abs2/1
  Saturation2/1 -> Gain2/1, Relay/1, WheelSpeed_rad/s/1
  Relay/1 -> Switch/2

== system xEMU_SimulationModel3_rule1/Drive Train (DRT)/Slipmodel and Traction /Variant Subsystem1/Mit_Schlupf_nach_Yoshiki/Slip Model ==
  note: Tangential Force Fx=Fz*u
      |
      | friction coefficient u=c*exp(-a*s)-d*exp(-b*s)
  Fz_tire : Inport
  slip_speed : Inport  Port=2
  adhesionCoefficient_abs : Inport  Port=3
  wheelspeed : Inport  Port=4
  " " : Fcn  Expr=1*exp(-0.54*u(1))-1*exp(-1.2*u(1))
  MATLAB Function1 : MATLAB Function  TreatAsAtomicUnit=on
  Product : Product
  Scope : Scope
  f_traction_tire : Outport
  wires:
  " "/1 -> MATLAB Function1/1(ad_factor)
  Fz_tire/1 -> Product/1
  slip_speed/1 -> " "/1
  [v_ist] -> MATLAB Function1/4(v_ist)
  [v_soll] -> MATLAB Function1/5(v_soll)
  Product/1 -> f_traction_tire/1
  adhesionCoefficient_abs/1 -> MATLAB Function1/2(ad_rail)
  MATLAB Function1/1(ad_factor_final) -> Product/2
  wheelspeed/1 -> Scope/1, MATLAB Function1/3(w)

== system xEMU_SimulationModel3_rule1/Drive Train (DRT)/Slipmodel and Traction /Variant Subsystem1/Mit_Schlupf_nach_Yoshiki/Tire Dynamics ==
  note: w
  Resistance of tire : Inport
  T_EMAdemandper_axis_Nm : Inport  Port=2
  v_train_m/s : Inport  Port=3
  Abs1 : Abs
  Abs2 : Abs
  Constant : Constant  Value=eps
  Gain : Gain  Gain=1/2
  Gain1 : Gain  Gain=1/J_drt
  Gain2 : Gain  Gain=R_wheel_drt_m
  Integrator : Integrator  LimitOutput=on  LowerSaturationLimit=0
  MATLAB Function : MATLAB Function  TreatAsAtomicUnit=on
  MATLAB Function1 : MATLAB Function  TreatAsAtomicUnit=on
  Max : MinMax  Function=max  Inputs=3
  Saturation : Saturate  UpperLimit=1  LowerLimit=-1
  Subtract : Sum  Inputs=+-
  Sum : Sum  Inputs=-+|
  slip : Scope
  slip_speed : Outport
  WheelSpeed_rad/s : Outport  Port=2
  wires:
  MATLAB Function/1(s) -> Saturation/1
  Constant/1 -> Max/3
  Abs2/1 -> Max/2
  Abs1/1 -> Max/1
  Saturation/1 -> slip/1
  Sum/1 -> Gain1/1
  Max/1 -> MATLAB Function/2(v)
  Gain1/1 -> Integrator/1
  Gain2/1 -> Subtract/1, Abs1/1
  T_EMAdemandper_axis_Nm/1 -> Gain/1
  Gain/1 -> MATLAB Function1/1(T_dem_per_axis)
  v_train_m/s/1 -> Abs2/1, Subtract/2
  Subtract/1 -> slip_speed/1, MATLAB Function/1(dv)  "Kalker"
  [v_soll] -> MATLAB Function1/2(v_soll)
  MATLAB Function1/1(T_dem_per_axis_final) -> Sum/2
  Integrator/1 -> Gain2/1, WheelSpeed_rad/s/1
  Resistance of tire/1 -> Sum/1

== system xEMU_SimulationModel3_rule1/Energy Manager (EMA)/Kern von EMS/P_load_aver/Subsystem/traction_motor_kennfeldbasiert ==
  "M_corr " : Inport
  n : Inport  Port=2
  2-D Pv_motor : Lookup_n-D  BreakpointsForDimension1=DRT.motor.torquevector  BreakpointsForDimension2=DRT.motor.speedvector  Table=DRT.motor.Pv_motor  ExtrapMethod=Clip  UseLastTableValue=on  InternalRulePriority=Speed  RndMeth=Simplest  InputSameDT=on
  Add : Sum
  Gain10 : Gain  Gain=1/1000
  Gain2 : Gain  Gain=1/1000
  Gain4 : Gain  Gain=0.99
  Gain5 : Gain  Gain=0.99
  Gain8 : Gain  Gain=2*pi/60
  MATLAB Function1 : MATLAB Function  TreatAsAtomicUnit=on
  M_obergenze : Lookup_n-D  NumberOfTableDimensions=1  BreakpointsForDimension1=DRT.motor.speedvector  Table=DRT.motor.torque_obergrenze  InternalRulePriority=Speed  RndMeth=Simplest  InputSameDT=on
  M_untergenze : Lookup_n-D  NumberOfTableDimensions=1  BreakpointsForDimension1=DRT.motor.speedvector  Table=DRT.motor.torque_untergrenze  InternalRulePriority=Speed  RndMeth=Simplest  InputSameDT=on
  Product4 : Product
  Subsystem : Subsystem
  umrichter efficiency : MATLAB Function  TreatAsAtomicUnit=on
  "P_el_corr " : Outport
  wires:
  Gain10/1 -> Add/1
  Gain8/1 -> Product4/2
  Product4/1 -> Gain10/1
  Gain2/1 -> Add/2
  MATLAB Function1/1(M_ist) -> Product4/1, Subsystem/1(M), 2-D Pv_motor/1
  M_obergenze/1 -> Gain4/1
  M_untergenze/1 -> Gain5/1
  Gain4/1 -> MATLAB Function1/3(M_max)
  Gain5/1 -> MATLAB Function1/2(M_min)
  "M_corr "/1 -> MATLAB Function1/1(M_soll)
  n/1 -> Subsystem/3("n "), 2-D Pv_motor/2, Gain8/1, M_obergenze/1, M_untergenze/1
  Subsystem/1(Pv_motor) -> Gain2/1
  2-D Pv_motor/1 -> Subsystem/2("lookuptable_Pv ")
  Add/1 -> umrichter efficiency/1(u)
  umrichter efficiency/1(y) -> "P_el_corr "/1

== system xEMU_SimulationModel3_rule1/Train Dynamics (TRM)/Variant Subsystem/v_t_model/Driver1/Subsystem ==
  F_soll : Inport
  v_train_ist : Inport  Port=2
  Add : Sum
  Divide : Product  Inputs=*/
  Divide1 : Product  Inputs=**
  Divide2 : Product  Inputs=**
  Gain1 : Gain  Gain=DRT.motor.gearratio_drt/DRT.slipmodel.R_wheel_drt_m
  Gain2 : Gain  Gain=1/DRT.slipmodel.R_wheel_drt_m
  Gain3 : Gain  Gain=DRT.slipmodel.R_wheel_drt_m/DRT.motor.gearratio_drt
  Gain4 : Gain  Gain=0.99
  Gain5 : Gain  Gain=0.99
  Gain6 : Gain  Gain=DRT.motor.gearratio_drt/DRT.slipmodel.R_wheel_drt_m
  Gain7 : Gain  Gain=DRT.motor.gearratio_drt*60/2/pi
  MATLAB Function1 : MATLAB Function  TreatAsAtomicUnit=on
  MATLAB Function2 : MATLAB Function  TreatAsAtomicUnit=on
  MATLAB Function3 : MATLAB Function  TreatAsAtomicUnit=on
  M_obergenze : Lookup_n-D  NumberOfTableDimensions=1  BreakpointsForDimension1=speedvector  Table=torque_obergrenze  InternalRulePriority=Speed  RndMeth=Simplest  InputSameDT=on
  M_untergenze : Lookup_n-D  NumberOfTableDimensions=1  BreakpointsForDimension1=speedvector  Table=torque_untergrenze  InternalRulePriority=Speed  RndMeth=Simplest  InputSameDT=on
  Out1 : Outport
  tag scope: F_EMA_min=global
  wires:
  v_train_ist/1 -> Gain2/1
  Divide1/1 -> Add/2
  Gain5/1 -> Gain1/1, MATLAB Function1/2(M_min)
  Gain4/1 -> MATLAB Function1/3(M_max)
  M_untergenze/1 -> Gain5/1
  M_obergenze/1 -> Gain4/1
  [num_EM] -> Divide/2, Divide1/1
  Gain3/1 -> Divide/1
  Divide/1 -> MATLAB Function1/1(M_soll)
  MATLAB Function1/1(M_ist) -> Gain6/1
  Gain2/1 -> Gain7/1
  Gain7/1 -> M_untergenze/1, M_obergenze/1
  MATLAB Function2/2(f_brake) -> Add/1
  Gain6/1 -> Divide1/2
  F_soll/1 -> MATLAB Function3/1(f_soll), MATLAB Function2/1(u)
  MATLAB Function3/1(f_actual) -> Out1/1
  MATLAB Function2/1(F_em) -> Gain3/1
  Add/1 -> MATLAB Function3/2(f_can)
  Gain1/1 -> Divide2/1
  [num_EM] -> Divide2/2
  Divide2/1 -> [F_EMA_min]

== system xEMU_SimulationModel3_rule1/Battery (BAT)_mittel/Battery/ElectricalCircuit/SerialTwoPort_Elem1/Cellelement_Elem1/OhmicResistance_Elem4 ==
  T : Inport
  SoC : Inport  Port=2
  Object : Lookup_n-D  BreakpointsForDimension1=[10 25 35 45]  BreakpointsForDimension2=[0 1 2 3 4 5 6 7 8 9 10 11 12 13 14 15 16 17 18 19 20 21 22 23 24 25 26 27 28 29 30 31 32 33 34 35 36 37 38 39 40 41 42 43 44 45 46 47 48 49 50 51 52 53 54 55 56 57 58 59 60 61 62 63 64 65 66 67 68 69 70 71 72 73 74 75 76 77 78 79 80 81 82 83 84 85 86 87 88 89 90 91 92 93 94 95 96 97 98 99 100]  Table=[0.00067277 0.00067277 0.00067277 0.00066956 0.00066636 0.00066316 0.00065995 0.00065675 0.00065395 0.0006513 0.00064864 0.00064598 0.00064333 0.00064066 0.000638 0.00063534 0.00063267 0.00063001 0.00062745 0.00062491 0.00062237 0.00061983 0.00061728 0.00061484 0.00061239 0.00060995 0.00060751 0.00060507 0.00060278 0.0006005 0.00059823 0.00059595 0.00059368 0.00059164 0.00058962 0.0005876 0.00058558 0.00058356 0.00058154 0.00057953 0.00057752 0.00057551 0.00057349 0.00057151 0.00056953 0.00056755 0.00056558 0.0005636 0.00056173 0.00055987 0.00055802 0.00055617 0.00055432 0.00055249 0.00055067 0.00054884 0.00054702 0.0005452 0.00054328 0.00054132 0.00053936 0.0005374 0.00053544 0.00053363 0.00053197 0.00053032 0.00052867 0.00052702 0.0005253 0.00052348 0.00052167 0.00051985 0.00051804 0.0005163 0.00051461 0.00051292 0.00051123 0.00050954 0.00050794 0.00050643 0.00050491 0.00050339 0.00050188 0.00050048 0.00049921 0.00049794 0.00049667 0.0004954 0.00049429 0.00049339 0.00049249 0.00049159 0.00049069 0.00048992 0.00048933 0.00048874 0.00048816 0.00048757 0.00048653 0.00048486 0.00048319;0.00067277 0.00067277 0.00067277 0.00066956 0.00066636 0.00066316 0.00065995 0.00065675 0.00065395 0.0006513 0.00064864 0.00064598 0.00064333 0.00064066 0.000638 0.00063534 0.00063267 0.00063001 0.00062745 0.00062491 0.00062237 0.00061983 0.00061728 0.00061484 0.00061239 0.00060995 0.00060751 0.00060507 0.00060278 0.0006005 0.00059823 0.00059595 0.00059368 0.00059164 0.00058962 0.0005876 0.00058558 0.00058356 0.00058154 0.00057953 0.00057752 0.00057551 0.00057349 0.00057151 0.00056953 0.00056755 0.00056558 0.0005636 0.00056173 0.00055987 0.00055802 0.00055617 0.00055432 0.00055249 0.00055067 0.00054884 0.00054702 0.0005452 0.00054328 0.00054132 0.00053936 0.0005374 0.00053544 0.00053363 0.00053197 0.00053032 0.00052867 0.00052702 0.0005253 0.00052348 0.00052167 0.00051985 0.00051804 0.0005163 0.00051461 0.00051292 0.00051123 0.00050954 0.00050794 0.00050643 0.00050491 0.00050339 0.00050188 0.00050048 0.00049921 0.00049794 0.00049667 0.0004954 0.00049429 0.00049339 0.00049249 0.00049159 0.00049069 0.00048992 0.00048933 0.00048874 0.00048816 0.00048757 0.00048653 0.00048486 0.00048319;0.00067277 0.00067277 0.00067277 0.00066956 0.00066636 0.00066316 0.00065995 0.00065675 0.00065395 0.0006513 0.00064864 0.00064598 0.00064333 0.00064066 0.000638 0.00063534 0.00063267 0.00063001 0.00062745 0.00062491 0.00062237 0.00061983 0.00061728 0.00061484 0.00061239 0.00060995 0.00060751 0.00060507 0.00060278 0.0006005 0.00059823 0.00059595 0.00059368 0.00059164 0.00058962 0.0005876 0.00058558 0.00058356 0.00058154 0.00057953 0.00057752 0.00057551 0.00057349 0.00057151 0.00056953 0.00056755 0.00056558 0.0005636 0.00056173 0.00055987 0.00055802 0.00055617 0.00055432 0.00055249 0.00055067 0.00054884 0.00054702 0.0005452 0.00054328 0.00054132 0.00053936 0.0005374 0.00053544 0.00053363 0.00053197 0.00053032 0.00052867 0.00052702 0.0005253 0.00052348 0.00052167 0.00051985 0.00051804 0.0005163 0.00051461 0.00051292 0.00051123 0.00050954 0.00050794 0.00050643 0.00050491 0.00050339 0.00050188 0.00050048 0.00049921 0.00049794 0.00049667 0.0004954 0.00049429 0.00049339 0.00049249 0.00049159 0.00049069 0.00048992 0.00048933 0.00048874 0.00048816 0.00048757 0.00048653 0.00048486 0.00048319;0.00067277 0.00067277 0.00067277 0.00066956 0.00066636 0.00066316 0.00065995 0.00065675 0.00065395 0.0006513 0.00064864 0.00064598 0.00064333 0.00064066 0.000638 0.00063534 0.00063267 0.00063001 0.00062745 0.00062491 0.00062237 0.00061983 0.00061728 0.00061484 0.00061239 0.00060995 0.00060751 0.00060507 0.00060278 0.0006005 0.00059823 0.00059595 0.00059368 0.00059164 0.00058962 0.0005876 0.00058558 0.00058356 0.00058154 0.00057953 0.00057752 0.00057551 0.00057349 0.00057151 0.00056953 0.00056755 0.00056558 0.0005636 0.00056173 0.00055987 0.00055802 0.00055617 0.00055432 0.00055249 0.00055067 0.00054884 0.00054702 0.0005452 0.00054328 0.00054132 0.00053936 0.0005374 0.00053544 0.00053363 0.00053197 0.00053032 0.00052867 0.00052702 0.0005253 0.00052348 0.00052167 0.00051985 0.00051804 0.0005163 0.00051461 0.00051292 0.00051123 0.00050954 0.00050794 0.00050643 0.00050491 0.00050339 0.00050188 0.00050048 0.00049921 0.00049794 0.00049667 0.0004954 0.00049429 0.00049339 0.00049249 0.00049159 0.00049069 0.00048992 0.00048933 0.00048874 0.00048816 0.00048757 0.00048653 0.00048486 0.00048319]  ExtrapMethod=Clip  RndMeth=Simplest  InputSameDT=on
  tag scope: ID2_ObjR=scoped
  wires:
  Object/1 -> [ID2_ObjR]
  T/1 -> Object/1
  SoC/1 -> Object/2
